simulink model "OPEN_LOOP_HINF_2020b_students"  (R2022b)
settings: Solver=VariableStepAuto  StartTime=0.0  StopTime=160  RelTol=1e-3  EnableMultiTasking=on
undefined symbols (not defined in the file or in its folder): delta, InitCond, model, omega, omegan, sys_osc_neust, sys_osc_unst
settings Model: Creator=croos  LastModifiedBy=fades
settings SolverCC: AlgebraicLoopSolver=TrustRegion
settings DataIOCC: LimitDataPoints=on  ReturnWorkspaceOutputs=off
settings OptimizationCC: LifeSpan=inf
settings DebuggingCC: AlgebraicLoopMsg=none  UnconnectedInputMsg=warning  UnconnectedOutputMsg=warning  UnconnectedLineMsg=warning  AllowSymbolicDim=off  SFUnexpectedBacktrackingDiag=warning  SFNoUnconditionalDefaultTransitionDiag=warning  SFExecutionAtInitializationDiag=none  SFMachineParentedDataDiag=warning  ArithmeticOperatorsInVariantConditions=warning
settings ModelReferenceCC: EnableRefExpFcnMdlSchedulingChecks=on  PropagateSignalLabelsOutOfModel=off
settings SFSimCC: SimUseLocalCustomCode=off  CustomCodeUndefinedFunction=UseInterfaceOnly
settings RTWCC: RTWUseLocalCustomCode=off  DLArmComputeVersion=19.05
settings CodeAppCC: StateflowObjectComments=on
settings GRTTargetCC: TargetLangStandard=C89/C90 (ANSI)
settings ConfigComp: CovMetricSettings=dw  CovSaveCumulativeToWorkspaceVar=on  CovSaveSingleToWorkspaceVar=on  CovExternalEMLEnable=off

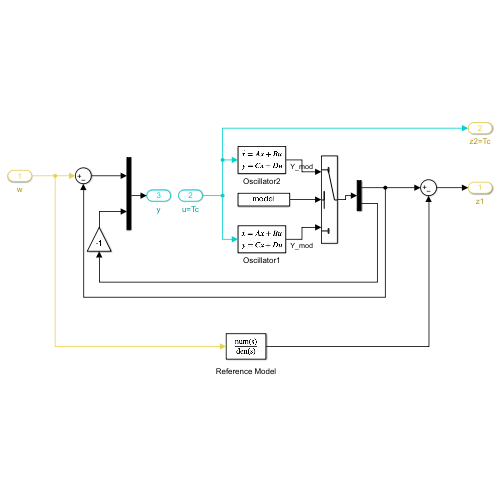
[thumbnail: Simulink's stored preview of the top-level diagram]
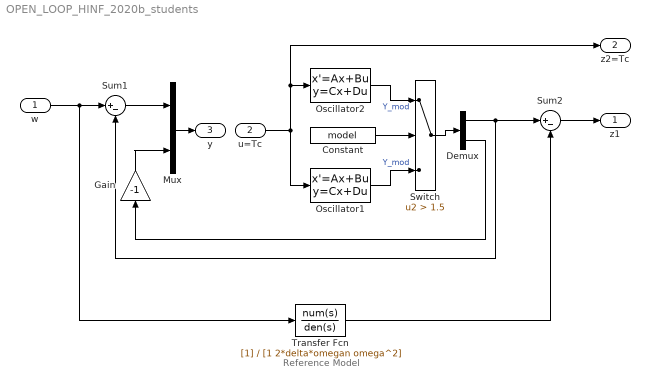
== system OPEN_LOOP_HINF_2020b_students ==
  note: Reference Model
  w : Inport
  u=Tc : Inport  Port=2
  Constant : Constant  Value=model
  Demux : Demux  Outputs=2
  Gain : Gain  Gain=-1
  Mux : Mux  Inputs=2
  Oscillator1 : StateSpace  A=sys_osc_unst.a  B=sys_osc_unst.b  C=sys_osc_unst.c  D=sys_osc_unst.d  InitialCondition=InitCond
  Oscillator2 : StateSpace  A=sys_osc_neust.a  B=sys_osc_neust.b  C=sys_osc_neust.c  D=sys_osc_neust.d  InitialCondition=InitCond
  Sum1 : Sum  Inputs=|+-
  Sum2 : Sum  Inputs=|+-
  Switch : Switch  Criteria=u2 > Threshold  Threshold=1.5  SaturateOnIntegerOverflow=off  InputSameDT=off
  Transfer Fcn : TransferFcn  Denominator=[1 2*delta*omegan omega^2]
  z1 : Outport
  z2=Tc : Outport  Port=2
  y : Outport  Port=3
  wires:
  Demux/1 -> Sum1/2, Sum2/1
  u=Tc/1 -> Oscillator1/1, Oscillator2/1, z2=Tc/1
  w/1 -> Transfer Fcn/1, Sum1/1
  Demux/2 -> Gain/1
  Mux/1 -> y/1
  Sum2/1 -> z1/1
  Transfer Fcn/1 -> Sum2/2
  Oscillator2/1 -> Switch/1  "Y_mod"
  Sum1/1 -> Mux/1
  Gain/1 -> Mux/2
  Oscillator1/1 -> Switch/3  "Y_mod"
  Switch/1 -> Demux/1
  Constant/1 -> Switch/2
